simulink model "Diesel_Genset_Test_System_80kVA"  (Simulink 8.1)
settings: Solver=ode3  SolverMode=SingleTasking  StartTime=0.0  StopTime=30  FixedStep=Ts  RelTol=1e-3
PostLoadFcn:
  | Ts=50e-6;GenSelect='80kW';initGTS;
InitFcn:
  | Ts=50e-6;GenSelect='80kW';initGTS;
values from neighbouring files (symbols this model uses):
  GenPN = 4e6    (= 4000000)    [initGTS.m]
  GenVN = 13800    [initGTS.m]
  T3dend = [ 1.0000   -0.9913 ]    [initGTS.m]
  T3numd = [ 0    0.0087 ]    [initGTS.m]
  T4numd = [ 27.7778  -27.7237 ]    [initGTS.m]
undefined symbols (not defined in the file or in its folder): breakers_1ph_3ph, Diesel_Genset_lib, DiscIntNeverNeededParam, Gen_900kW_external_control, HIL_GenSet, Protection
libraries: powerlib x41, simulink x20, powerlib_extras x12, NG_Genset_lib x5, rtlab x2, cables_lib x2, powerlib_meascontrol x1
(part 2 of 2)

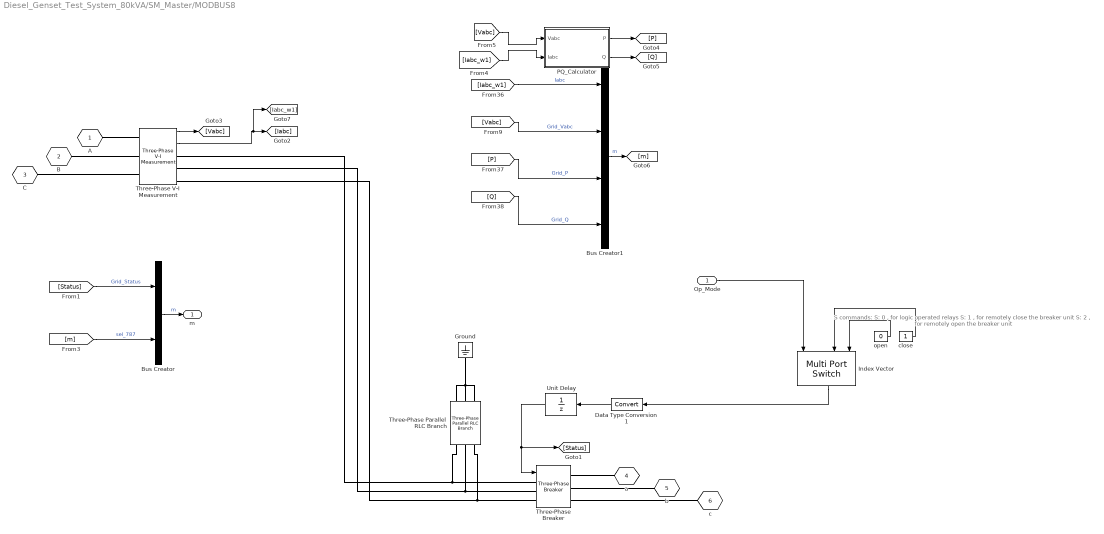
== system Diesel_Genset_Test_System_80kVA/SM_Master/MODBUS8 ==
  note: S commands:
      | S: 0 , for logic operated relays
      | S: 1 ,  for remotely close the breaker unit
      | S: 2 , for remotely open the breaker unit
  Op_Mode : Inport
  Bus Creator : BusCreator  Inputs=2
  Bus Creator1 : BusCreator
  Data Type Conversion1 : DataTypeConversion
  Ground : powerlib/Elements/Ground  LConnTagsString=a
  Index Vector : MultiPortSwitch  DataPortOrder=Zero-based contiguous  DataPortIndices={2,1,0}  zeroidx=on
  PQ_Calculator : Subsystem
  Three-Phase Parallel RLC Branch : powerlib/Elements/Three-Phase Parallel RLC Branch  LConnTagsString=A|B|C  RConnTagsString=A|B|C  BranchType=R  Resistance=10e6  Inductance=1e-3  Capacitance=1e-6  Measurements=None
  Three-Phase V-I Measurement : powerlib/Measurements/Three-Phase V-I Measurement  VoltageMeasurement=phase-to-ground  SetLabelV=off  LabelV=Vabc  Vpu=off  VpuLL=off  CurrentMeasurement=yes  SetLabelI=off  LabelI=Iabc  Ipu=off  Pbase=100e6  Vbase=500e3  OutputType=Complex  PhasorSimulation=off  PSBequivalent=0
  Three-Phase Breaker : powerlib/Elements/Three-Phase Breaker  InitialState=open  SwitchA=on  SwitchB=on  SwitchC=on  SwitchTimes="[1/60  5/60]"  External=on  BreakerResistance=1e-3  SnubberResistance=0  SnubberCapacitance=0  Measurements=None
  Unit Delay : UnitDelay  SampleTime=-1
  close : Constant
  open : Constant  Value=0
  A : PMIOPort  Tag=PMCPort  Port=1  Side=Left
  B : PMIOPort  Tag=PMCPort  Port=2  Side=Left
  C : PMIOPort  Tag=PMCPort  Port=3  Side=Left
  a : PMIOPort  Tag=PMCPort  Port=4  Side=Right
  b : PMIOPort  Tag=PMCPort  Port=5  Side=Right
  c : PMIOPort  Tag=PMCPort  Port=6  Side=Right
  m : Outport
  wires:
  [m] -> Bus Creator/2  "sel_787"
  Bus Creator/1 -> m/1  "m"
  [Status] -> Bus Creator/1  "Grid_Status"
  Unit Delay/1 -> [Status], Three-Phase Breaker/1
  Three-Phase V-I Measurement/1 -> [Vabc]
  Three-Phase V-I Measurement/2 -> [Iabc_w1], [Iabc]
  open/1 -> Index Vector/4
  close/1 -> Index Vector/3
  Index Vector/1 -> Data Type Conversion1/1
  Data Type Conversion1/1 -> Unit Delay/1
  Op_Mode/1 -> Index Vector/1
  [Q] -> Bus Creator1/4  "Grid_Q"
  [P] -> Bus Creator1/3  "Grid_P"
  [Vabc] -> Bus Creator1/2  "Grid_Vabc"
  [Iabc_w1] -> Bus Creator1/1  "Iabc"
  Bus Creator1/1 -> [m]  "m"
  [Vabc] -> PQ_Calculator/1(Vabc)
  [Iabc_w1] -> PQ_Calculator/2(Iabc)
  PQ_Calculator/1(P) -> [P]
  PQ_Calculator/2(Q) -> [Q]
  connections:
  Three-Phase V-I Measurement/RConn1 -- Three-Phase Parallel RLC Branch/RConn1 -- Three-Phase Breaker/LConn1
  Three-Phase V-I Measurement/RConn2 -- Three-Phase Parallel RLC Branch/RConn2 -- Three-Phase Breaker/LConn2
  Three-Phase V-I Measurement/RConn3 -- Three-Phase Parallel RLC Branch/RConn3 -- Three-Phase Breaker/LConn3
  Three-Phase Breaker/RConn2 -- b/RConn1
  Three-Phase Breaker/RConn3 -- c/RConn1
  Three-Phase V-I Measurement/LConn1 -- A/RConn1
  a/RConn1 -- Three-Phase Breaker/RConn1
  C/RConn1 -- Three-Phase V-I Measurement/LConn3
  B/RConn1 -- Three-Phase V-I Measurement/LConn2
  Ground/LConn1 -- Three-Phase Parallel RLC Branch/LConn2 -- Three-Phase Parallel RLC Branch/LConn3 -- Three-Phase Parallel RLC Branch/LConn1

== system Diesel_Genset_Test_System_80kVA/SC_Console/Woodward/16Din/16Dout GR3 ==
  Bus Creator2 : BusCreator  Inputs=8
  Closed 3 - 26 s1 : simulink/Sources/Repeating Sequence Stair  OutValues=[1 1 1 0 0 0 0 0 0 0 0 0 0 0 0 0 0 0 0 0 0 0 0 0 0 0 1 1 1 1 1 ]  tsamp=[1 Ts]  OutMin=[]  OutMax=[]  OutDataTypeStr=double  OutputDataTypeScalingMode=double  OutDataType=fixdt(0,8)  ConRadixGroup=Best Precision: Vector-wise  OutScaling=2^-12
  Constant5 : Constant  Value=0
  Constant6 : Constant
  Constant7 : Constant  Value=0
  Constant8 : Constant
  DO10_ExtAlarm : ManualSwitch  CurrentSetting=0
  DO11_EnableMCB : ManualSwitch  CurrentSetting=0
  DO12_MCBOpen : ManualSwitch  CurrentSetting=0
  DO13_GCBOpen : ManualSwitch  CurrentSetting=0
  DO14 : ManualSwitch  CurrentSetting=0
  DO15 : ManualSwitch  CurrentSetting=0
  DO8_Estop : ManualSwitch
  DO9_Start/Auto : ManualSwitch  CurrentSetting=0
  Dout : Outport
  wires:
  Bus Creator2/1 -> Dout/1  "DO"
  Constant6/1 -> DO9_Start/Auto/1, DO11_EnableMCB/1, DO10_ExtAlarm/1, DO8_Estop/1
  Constant5/1 -> DO9_Start/Auto/2, DO11_EnableMCB/2, DO10_ExtAlarm/2, DO8_Estop/2
  DO8_Estop/1 -> Bus Creator2/1  "Gen_Estop"
  DO9_Start/Auto/1 -> Bus Creator2/2  "Gen_StartAuto"
  DO10_ExtAlarm/1 -> Bus Creator2/3  "Gen_ExtAlarm"
  DO11_EnableMCB/1 -> Bus Creator2/4  "Gen_EnableMCB"
  Constant8/1 -> DO14/1, DO15/1, DO13_GCBOpen/1, DO12_MCBOpen/1
  Constant7/1 -> DO14/2, DO15/2, DO13_GCBOpen/2, DO12_MCBOpen/2
  DO12_MCBOpen/1 -> Bus Creator2/5  "Gen_MCBOpen"
  DO14/1 -> Bus Creator2/7  "Gen_DI11_MCB_Busbar"
  DO15/1 -> Bus Creator2/8  "Gen_DI12_GCB_Busbar"
  Closed 3 - 26 s1/1 -> Bus Creator2/6  "Gen_GCBOpen"

== system Diesel_Genset_Test_System_80kVA/SM_Master/80kVA_Diesel_Generator/DIO - Woodward ==
  note: These are the inputs to
      | Woodward
  Din_sim : Inport
  Gen2 MCB Status : Inport  Port=2
  Add2 : Sum
  Bus Selector2 : BusSelector  OutputSignals=Gen_Estop,Gen_StartAuto,Gen_ExtAlarm,Gen_EnableMCB,Gen_MCBOpen,Gen_GCBOpen,Gen_DI11_MCB_Busbar,Gen_DI12_GCB_Busbar
  Constant3 : Constant
  Data Type Conversion : DataTypeConversion  OutDataTypeStr=double
  Logical Operator1 : Logic  Operator=NOT  AllPortsSameDT=off  OutDataTypeStr=boolean
  Mux1 : Mux  Inputs=8
  Gen2 GCB : Outport
  wires:
  Mux1/1 -> ?  "DI_CH08-15"
  Add2/1 -> Gen2 GCB/1
  Constant3/1 -> Add2/2
  Bus Selector2/1 -> Mux1/1  "<Gen_Estop>"
  Bus Selector2/2 -> Mux1/2  "<Gen_StartAuto>"
  Bus Selector2/3 -> Mux1/3  "<Gen_ExtAlarm>"
  Bus Selector2/4 -> Mux1/4  "<Gen_EnableMCB>"
  Bus Selector2/5 -> ?  "<Gen_MCBOpen>"
  Bus Selector2/6 -> Add2/1, Mux1/6  "<Gen_GCBOpen>"
  Din_sim/1 -> Bus Selector2/1
  Bus Selector2/7 -> ?  "<Gen_DI11_MCB_Busbar>"
  Gen2 MCB Status/1 -> Mux1/7, Logical Operator1/1
  Bus Selector2/8 -> Mux1/8  "<Gen_DI12_GCB_Busbar>"
  Logical Operator1/1 -> Data Type Conversion/1
  Data Type Conversion/1 -> Mux1/5

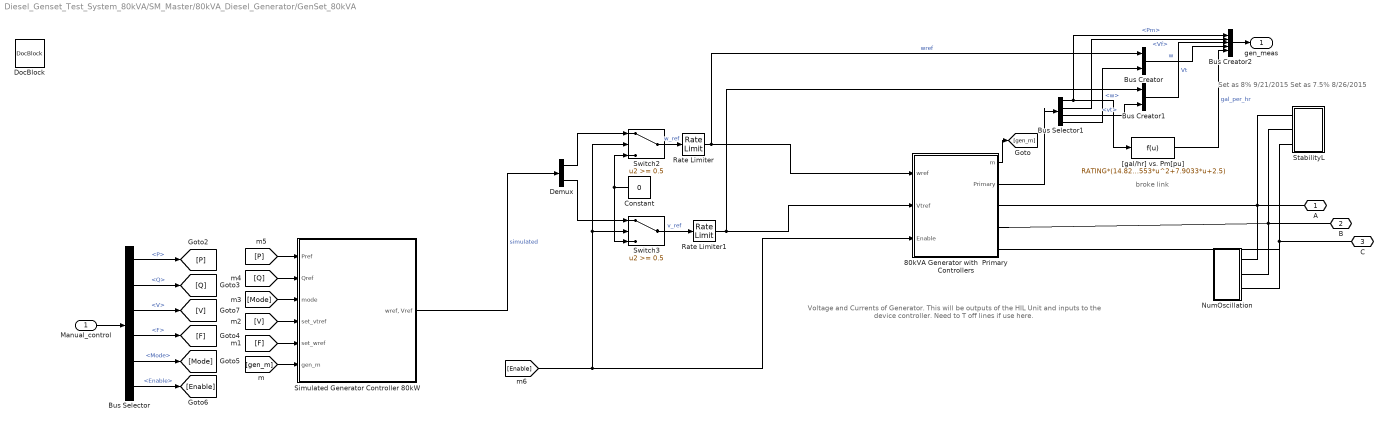
== system Diesel_Genset_Test_System_80kVA/SM_Master/80kVA_Diesel_Generator/GenSet_80kVA ==
  note: broke link
  note: Set as 8% 9/21/2015
      | Set as 7.5% 8/26/2015
  note: Voltage and Currents of Generator.
      | This will be outputs of the HIL Unit
      | and inputs to the device controller.
      | Need to T off lines if use here.
  Manual_control : Inport
  80kVA Generator with  Primary Controllers : Subsystem
  Bus Creator : BusCreator  Inputs=2
  Bus Creator1 : BusCreator  Inputs=2
  Bus Creator2 : BusCreator  Inputs=5
  Bus Selector : BusSelector  OutputSignals=P,Q,V,F,Mode,Enable
  Bus Selector1 : BusSelector  OutputSignals=Pm,Vf,vt,w
  Constant : Constant  Value=0
  Demux : Demux  Outputs=2
  DocBlock : simulink/Model-Wide Utilities/DocBlock  DocumentType=Text
  NumOscillation : Subsystem
  Rate Limiter : RateLimiter  RisingSlewLimit=0.5  FallingSlewLimit=-0.5  SampleTimeMode=inherited
  Rate Limiter1 : RateLimiter  RisingSlewLimit=0.5  FallingSlewLimit=-0.5  SampleTimeMode=inherited
  Simulated Generator Controller 80kW : Subsystem
  StabilityL : Subsystem  mask{v=GenVN, kVA=GenPN*0.2/1000, pf=1}
  Switch2 : Switch  Threshold=0.5
  Switch3 : Switch  Threshold=0.5
  "[gal/hr] vs. Pm[pu]" : Fcn  Expr=RATING*(14.827*u^4-27.253*u^3+15.553*u^2+7.9033*u+2.5)  mask{RATING=4}
      mask prompts: RATING "Rating [MW]"
      mask help: This block computes the gal/hr vs Pm[pu] of a generator of a given rating [MW].
  A : PMIOPort  Port=1  Side=Right
  B : PMIOPort  Port=2  Side=Right
  C : PMIOPort  Port=3  Side=Right
  gen_meas : Outport
  wires:
  "[gal/hr] vs. Pm[pu]"/1 -> Bus Creator2/5  "gal_per_hr"
  Rate Limiter1/1 -> Bus Creator1/1, 80kVA Generator with  Primary Controllers/2(Vtref)
  Rate Limiter/1 -> Bus Creator/1, 80kVA Generator with  Primary Controllers/1(wref)  "wref"
  Bus Creator2/1 -> gen_meas/1
  Bus Creator/1 -> Bus Creator2/4  "w"
  Bus Creator1/1 -> Bus Creator2/3  "Vt"
  Bus Selector1/1 -> "[gal/hr] vs. Pm[pu]"/1, Bus Creator2/1  "<Pm>"
  Bus Selector1/2 -> Bus Creator2/2  "<Vf>"
  Bus Selector1/4 -> Bus Creator/2  "<w>"
  Bus Selector1/3 -> Bus Creator1/2  "<vt>"
  Switch3/1 -> Rate Limiter1/1  "v_ref"
  Constant/1 -> Switch2/3, Switch3/3
  Demux/2 -> Switch3/1
  Demux/1 -> Switch2/1
  Switch2/1 -> Rate Limiter/1  "w_ref"
  [Enable] -> Switch3/2, Switch2/2, 80kVA Generator with  Primary Controllers/3(Enable)
  80kVA Generator with  Primary Controllers/2(Primary) -> Bus Selector1/1
  Bus Selector/6 -> [Enable]  "<Enable>"
  80kVA Generator with  Primary Controllers/1(m) -> [gen_m]
  Simulated Generator Controller 80kW/1("wref, Vref") -> Demux/1  "simulated"
  Manual_control/1 -> Bus Selector/1
  Bus Selector/1 -> [P]  "<P>"
  Bus Selector/2 -> [Q]  "<Q>"
  Bus Selector/3 -> [V]  "<V>"
  Bus Selector/4 -> [F]  "<F>"
  Bus Selector/5 -> [Mode]  "<Mode>"
  [gen_m] -> Simulated Generator Controller 80kW/6(gen_m)
  [P] -> Simulated Generator Controller 80kW/1(Pref)
  [Q] -> Simulated Generator Controller 80kW/2(Qref)
  [Mode] -> Simulated Generator Controller 80kW/3(mode)
  [V] -> Simulated Generator Controller 80kW/4(set_vtref)
  [F] -> Simulated Generator Controller 80kW/5(set_wref)
  connections:
  NumOscillation/LConn3 -- 80kVA Generator with  Primary Controllers/RConn3 -- C/RConn1 -- StabilityL/LConn3
  NumOscillation/LConn2 -- B/RConn1 -- 80kVA Generator with  Primary Controllers/RConn2 -- StabilityL/LConn2
  NumOscillation/LConn1 -- 80kVA Generator with  Primary Controllers/RConn1 -- A/RConn1 -- StabilityL/LConn1

== system Diesel_Genset_Test_System_80kVA/SM_Master/MODBUS1/PQ_Calculator ==
  Vabc : Inport
  Iabc : Inport  Port=2
  3-phase  Instantaneous  Active & Reactive Power : powerlib_extras/Measurements/3-phase  Instantaneous  Active & Reactive Power
  Demux : Demux  Outputs=2
  Discrete  Mean value2 : powerlib_extras/Discrete Measurements/Discrete  Mean value  Freq=60  Vinit=0  Ts=Ts
  P : Outport
  Q : Outport  Port=2
  wires:
  3-phase  Instantaneous  Active & Reactive Power/1 -> Discrete  Mean value2/1
  Discrete  Mean value2/1 -> Demux/1
  Vabc/1 -> 3-phase  Instantaneous  Active & Reactive Power/1
  Iabc/1 -> 3-phase  Instantaneous  Active & Reactive Power/2
  Demux/1 -> P/1  "P"
  Demux/2 -> Q/1  "Q"

== system Diesel_Genset_Test_System_80kVA/SM_Master/MODBUS2/PQ_Calculator ==
  Vabc : Inport
  Iabc : Inport  Port=2
  3-phase  Instantaneous  Active & Reactive Power : powerlib_extras/Measurements/3-phase  Instantaneous  Active & Reactive Power
  Demux : Demux  Outputs=2
  Discrete  Mean value2 : powerlib_extras/Discrete Measurements/Discrete  Mean value  Freq=60  Vinit=0  Ts=Ts
  P : Outport
  Q : Outport  Port=2
  wires:
  3-phase  Instantaneous  Active & Reactive Power/1 -> Discrete  Mean value2/1
  Discrete  Mean value2/1 -> Demux/1
  Vabc/1 -> 3-phase  Instantaneous  Active & Reactive Power/1
  Iabc/1 -> 3-phase  Instantaneous  Active & Reactive Power/2
  Demux/1 -> P/1  "P"
  Demux/2 -> Q/1  "Q"

== system Diesel_Genset_Test_System_80kVA/SM_Master/MODBUS4/PQ_Calculator ==
  Vabc : Inport
  Iabc : Inport  Port=2
  3-phase  Instantaneous  Active & Reactive Power : powerlib_extras/Measurements/3-phase  Instantaneous  Active & Reactive Power
  Demux : Demux  Outputs=2
  Discrete  Mean value2 : powerlib_extras/Discrete Measurements/Discrete  Mean value  Freq=60  Vinit=0  Ts=Ts
  P : Outport
  Q : Outport  Port=2
  wires:
  3-phase  Instantaneous  Active & Reactive Power/1 -> Discrete  Mean value2/1
  Discrete  Mean value2/1 -> Demux/1
  Vabc/1 -> 3-phase  Instantaneous  Active & Reactive Power/1
  Iabc/1 -> 3-phase  Instantaneous  Active & Reactive Power/2
  Demux/1 -> P/1  "P"
  Demux/2 -> Q/1  "Q"

== system Diesel_Genset_Test_System_80kVA/SM_Master/MODBUS5/PQ_Calculator ==
  Vabc : Inport
  Iabc : Inport  Port=2
  3-phase  Instantaneous  Active & Reactive Power : powerlib_extras/Measurements/3-phase  Instantaneous  Active & Reactive Power
  Demux : Demux  Outputs=2
  Discrete  Mean value2 : powerlib_extras/Discrete Measurements/Discrete  Mean value  Freq=60  Vinit=0  Ts=Ts
  P : Outport
  Q : Outport  Port=2
  wires:
  3-phase  Instantaneous  Active & Reactive Power/1 -> Discrete  Mean value2/1
  Discrete  Mean value2/1 -> Demux/1
  Vabc/1 -> 3-phase  Instantaneous  Active & Reactive Power/1
  Iabc/1 -> 3-phase  Instantaneous  Active & Reactive Power/2
  Demux/1 -> P/1  "P"
  Demux/2 -> Q/1  "Q"

== system Diesel_Genset_Test_System_80kVA/SM_Master/MODBUS6/PQ_Calculator ==
  Vabc : Inport
  Iabc : Inport  Port=2
  3-phase  Instantaneous  Active & Reactive Power : powerlib_extras/Measurements/3-phase  Instantaneous  Active & Reactive Power
  Demux : Demux  Outputs=2
  Discrete  Mean value2 : powerlib_extras/Discrete Measurements/Discrete  Mean value  Freq=60  Vinit=0  Ts=Ts
  P : Outport
  Q : Outport  Port=2
  wires:
  3-phase  Instantaneous  Active & Reactive Power/1 -> Discrete  Mean value2/1
  Discrete  Mean value2/1 -> Demux/1
  Vabc/1 -> 3-phase  Instantaneous  Active & Reactive Power/1
  Iabc/1 -> 3-phase  Instantaneous  Active & Reactive Power/2
  Demux/1 -> P/1  "P"
  Demux/2 -> Q/1  "Q"

== system Diesel_Genset_Test_System_80kVA/SM_Master/MODBUS8/PQ_Calculator ==
  Vabc : Inport
  Iabc : Inport  Port=2
  3-phase  Instantaneous  Active & Reactive Power : powerlib_extras/Measurements/3-phase  Instantaneous  Active & Reactive Power
  Demux : Demux  Outputs=2
  Discrete  Mean value2 : powerlib_extras/Discrete Measurements/Discrete  Mean value  Freq=60  Vinit=0  Ts=Ts
  P : Outport
  Q : Outport  Port=2
  wires:
  3-phase  Instantaneous  Active & Reactive Power/1 -> Discrete  Mean value2/1
  Discrete  Mean value2/1 -> Demux/1
  Vabc/1 -> 3-phase  Instantaneous  Active & Reactive Power/1
  Iabc/1 -> 3-phase  Instantaneous  Active & Reactive Power/2
  Demux/1 -> P/1  "P"
  Demux/2 -> Q/1  "Q"

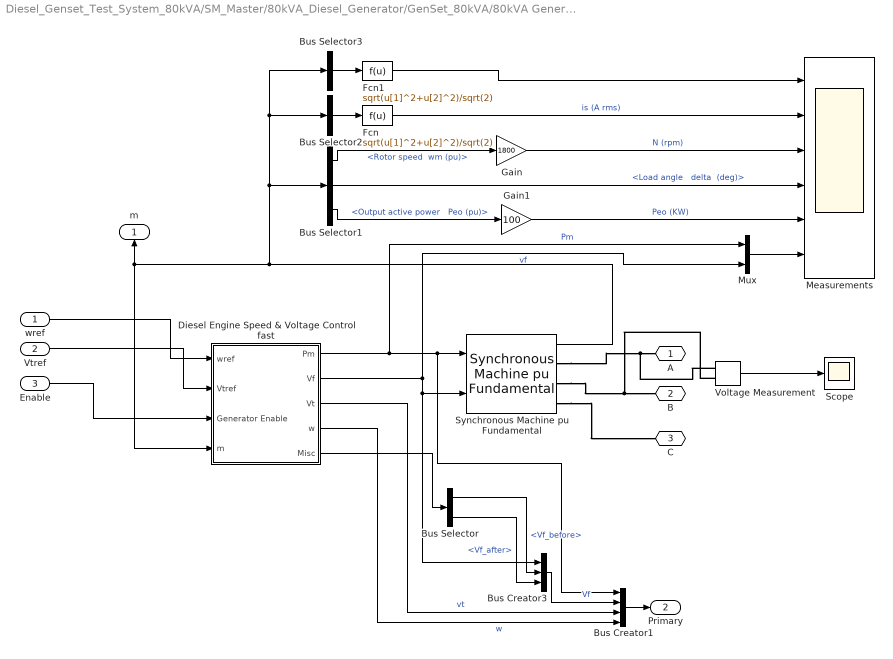
== system Diesel_Genset_Test_System_80kVA/SM_Master/80kVA_Diesel_Generator/GenSet_80kVA/80kVA Generator with  Primary Controllers ==
  wref : Inport
  Vtref : Inport  Port=2
  Enable : Inport  Port=3
  Bus Creator1 : BusCreator
  Bus Creator3 : BusCreator  Inputs=3
  Bus Selector : BusSelector  OutputSignals=Vf_before,Vf_after
  Bus Selector1 : BusSelector  OutputSignals="Mechanical.Rotor speed  wm (pu),Load angle   delta  (deg),Output active power   Peo (pu)"
  Bus Selector2 : BusSelector  OutputSignals="dq0 components.Stator current  iq (pu),dq0 components.Stator current  id (pu)"  OutputAsBus=on
  Bus Selector3 : BusSelector  OutputSignals="dq0 components.Stator voltage  vq (pu),dq0 components.Stator voltage  vd (pu)"  OutputAsBus=on
  Diesel Engine Speed & Voltage Control fast : Subsystem
  Fcn : Fcn  Expr=sqrt(u[1]^2+u[2]^2)/sqrt(2)
  Fcn1 : Fcn  Expr=sqrt(u[1]^2+u[2]^2)/sqrt(2)
  Gain : Gain  Gain=1800  SaturateOnIntegerOverflow=on  OutDataTypeStr=Inherit: Same as input  ParamDataTypeStr=Inherit: Same as input
  Gain1 : Gain  Gain=100  SaturateOnIntegerOverflow=on  OutDataTypeStr=Inherit: Same as input  ParamDataTypeStr=Inherit: Same as input
  Measurements : Scope  NumInputPorts=6
      settings: TickLabels=on  TimeRange=3  YMin=0.1~0~1500~-200~-400~-1  YMax=0.8~8~2100~200~300~5  SaveName=is
  Mux : Mux  Inputs=2
  Scope : Scope
      settings: YMin=-750  YMax=750  SaveName=ScopeData12  Decimation=10
  Synchronous Machine pu Fundamental : powerlib/Machines/Synchronous Machine pu Fundamental  PresetModel=No  MechanicalLoad=Mechanical power Pm  ShowDetailedParameters=on  RotorType=Salient-pole  NominalParameters=[80e3 480 60]  Stator=[0.02599 0.07 2.25 0.99]  Field=[0.016 0.2092]  Dampers2=[0.0652, 0.5134, 0.0287, 0.2553, 7.765e-3, 0.9167 ]  Dampers1=[0.2047 0.6524 0.04286 0.06387]  Mechanical=[0.1268 0.02132 2]  PolePairs=2  InitialConditions="[ -99  0  0  0  0  0  0  0  0 ]"  SetSaturation=off  Saturation=[0.6404,0.7127,0.8441,0.9214,0.9956,1.082,1.19,1.316,1.457;0.7,0.7698,0.8872,0.9466,0.9969,1.046,1.1,1.151,1.201]  Units=per unit fundamental parameters  LoadFlowParameters=[1,0,0,0,0]  TsPowergui=0  TsBlock=-1  IterativeModel=Forward Euler  BusType=swing  Pref=0  Qref=0  Qmin=-inf  Qmax=inf  PLF=0  QLF=0
  Voltage Measurement : powerlib/Measurements/Voltage Measurement  PhasorSimulation=off  OutputType=Complex  PSBequivalent=0
  A : PMIOPort  Port=1  Side=Right
  B : PMIOPort  Port=2  Side=Right
  C : PMIOPort  Port=3  Side=Right
  m : Outport
  Primary : Outport  Port=2
  wires:
  Bus Creator3/1 -> Bus Creator1/2  "Vf"
  Bus Selector/2 -> Bus Creator3/3  "<Vf_after>"
  Bus Selector/1 -> Bus Creator3/2  "<Vf_before>"
  Diesel Engine Speed & Voltage Control fast/5(Misc) -> Bus Selector/1
  Bus Creator1/1 -> Primary/1
  Diesel Engine Speed & Voltage Control fast/4(w) -> Bus Creator1/4  "w"
  Diesel Engine Speed & Voltage Control fast/3(Vt) -> Bus Creator1/3  "vt"
  Synchronous Machine pu Fundamental/1 -> Bus Selector1/1, Bus Selector2/1, Bus Selector3/1, Diesel Engine Speed & Voltage Control fast/4(m), m/1
  Enable/1 -> Diesel Engine Speed & Voltage Control fast/3(Generator Enable)
  Diesel Engine Speed & Voltage Control fast/1(Pm) -> Mux/1, Synchronous Machine pu Fundamental/1, Bus Creator1/1  "Pm"
  Diesel Engine Speed & Voltage Control fast/2(Vf) -> Synchronous Machine pu Fundamental/2, Bus Creator3/1, Mux/2  "vf"
  wref/1 -> Diesel Engine Speed & Voltage Control fast/1(wref)
  Vtref/1 -> Diesel Engine Speed & Voltage Control fast/2(Vtref)
  Fcn/1 -> Measurements/2  "is (A rms)"
  Bus Selector2/1 -> Fcn/1
  Gain/1 -> Measurements/3  "N (rpm)"
  Gain1/1 -> Measurements/5  "Peo (KW)"
  Bus Selector1/3 -> Gain1/1  "<Output active power   Peo (pu)>"
  Bus Selector1/2 -> Measurements/4  "<Load angle   delta  (deg)>"
  Bus Selector1/1 -> Gain/1  "<Rotor speed  wm (pu)>"
  Bus Selector3/1 -> Fcn1/1
  Fcn1/1 -> Measurements/1
  Mux/1 -> Measurements/6
  Voltage Measurement/1 -> Scope/1
  connections:
  Synchronous Machine pu Fundamental/RConn1 -- Voltage Measurement/LConn1 -- A/RConn1
  Synchronous Machine pu Fundamental/RConn2 -- Voltage Measurement/LConn2 -- B/RConn1
  Synchronous Machine pu Fundamental/RConn3 -- C/RConn1

== system Diesel_Genset_Test_System_80kVA/SM_Master/80kVA_Diesel_Generator/GenSet_80kVA/NumOscillation ==
  Ground2 : powerlib/Elements/Ground  LConnTagsString=a
  "RLC " : powerlib/Elements/Parallel RLC Branch  LConnTagsString=a  RConnTagsString=__new0  BranchType=R  Resistance=10e6  Inductance=inf  SetiL0=off  InitialCurrent=0  Capacitance=10e-6  Setx0=off  InitialVoltage=0  Measurements=None
  RLC1 : powerlib/Elements/Parallel RLC Branch  LConnTagsString=a  RConnTagsString=__new0  BranchType=R  Resistance=10e6  Inductance=inf  SetiL0=off  InitialCurrent=0  Capacitance=10e-6  Setx0=off  InitialVoltage=0  Measurements=None
  RLC2 : powerlib/Elements/Parallel RLC Branch  LConnTagsString=a  RConnTagsString=__new0  BranchType=R  Resistance=10e6  Inductance=inf  SetiL0=off  InitialCurrent=0  Capacitance=10e-6  Setx0=off  InitialVoltage=0  Measurements=None
  RLC3 : powerlib/Elements/Parallel RLC Branch  LConnTagsString=a  RConnTagsString=__new0  BranchType=R  Resistance=10e-3  Inductance=inf  SetiL0=off  InitialCurrent=0  Capacitance=0  Setx0=off  InitialVoltage=0  Measurements=None
  RLC4 : powerlib/Elements/Parallel RLC Branch  LConnTagsString=a  RConnTagsString=__new0  BranchType=R  Resistance=10e-3  Inductance=inf  SetiL0=off  InitialCurrent=0  Capacitance=0  Setx0=off  InitialVoltage=0  Measurements=None
  RLC5 : powerlib/Elements/Parallel RLC Branch  LConnTagsString=a  RConnTagsString=__new0  BranchType=R  Resistance=10e-3  Inductance=inf  SetiL0=off  InitialCurrent=0  Capacitance=0  Setx0=off  InitialVoltage=0  Measurements=None
  A : PMIOPort  Port=1  Side=Left
  B : PMIOPort  Port=2  Side=Left
  C : PMIOPort  Port=3  Side=Left
  connections:
  "RLC "/RConn1 -- RLC1/RConn1 -- Ground2/LConn1 -- RLC2/RConn1
  "RLC "/LConn1 -- RLC5/RConn1
  RLC1/LConn1 -- RLC4/RConn1
  RLC3/RConn1 -- RLC2/LConn1
  A/RConn1 -- RLC3/LConn1
  B/RConn1 -- RLC4/LConn1
  C/RConn1 -- RLC5/LConn1

== system Diesel_Genset_Test_System_80kVA/SM_Master/80kVA_Diesel_Generator/GenSet_80kVA/Simulated Generator Controller 80kW ==
  Pref : Inport
  Qref : Inport  Port=2
  mode : Inport  Port=3
  set_vtref : Inport  Port=4
  set_wref : Inport  Port=5
  gen_m : Inport  Port=6
  Bus Selector1 : BusSelector  OutputSignals="Output active power   Peo (pu),Output reactive power  Qeo (pu)"
  Compare To Constant : simulink/Logic and Bit Operations/Compare To Constant  relop=~=  const=1  OutDataTypeStr=boolean
  Demux : Demux  Outputs=2
  Multiport Switch : MultiPortSwitch  DiagnosticForDefault=Warning
  Mux1 : Mux  Inputs=2
  Mux2 : Mux  Inputs=2
  Mux3 : Mux  Inputs=2
  PQ control : Subsystem
  PV control : Subsystem
  Unit Delay : UnitDelay  SampleTime=-1
  "wref, Vref" : Outport
  wires:
  Multiport Switch/1 -> Unit Delay/1, "wref, Vref"/1
  mode/1 -> Compare To Constant/1, Multiport Switch/1
  Qref/1 -> PQ control/3(Q_ref (pu))
  set_wref/1 -> Mux3/1
  Bus Selector1/2 -> PQ control/4(Q (pu))  "<Output reactive power  Qeo (pu)>"
  Pref/1 -> PV control/1(P_ref (pu)), PQ control/1(P_ref (pu))
  Mux3/1 -> Multiport Switch/4
  Mux2/1 -> Multiport Switch/3
  Mux1/1 -> Multiport Switch/2
  set_vtref/1 -> Mux3/2, Mux2/2
  PV control/1(w_ref (pu)) -> Mux2/1
  PQ control/2(V_ref (pu)) -> Mux1/2
  PQ control/1(w_ref (pu)) -> Mux1/1
  gen_m/1 -> Bus Selector1/1
  Bus Selector1/1 -> PV control/2(P (pu)), PQ control/2(P (pu))  "<Output active power   Peo (pu)>"
  Compare To Constant/1 -> PQ control/5(Rst)
  Demux/1 -> PQ control/6(w_Rst)
  Demux/2 -> PQ control/7(V_Rst)
  Unit Delay/1 -> Demux/1

== system Diesel_Genset_Test_System_80kVA/SM_Master/80kVA_Diesel_Generator/GenSet_80kVA/StabilityL ==
  Constant Load : powerlib/Elements/Three-Phase Parallel RLC Load  LConnTagsString=A|B|C  Configuration=Y (grounded)  NominalVoltage=v  NominalFrequency=60  ActivePower=kVA*1E3*pf  InductivePower=kVA*1E3*sqrt(1-pf^2)  CapacitivePower=0  Measurements=None  LoadType=constant Z
  A : PMIOPort  Port=1  Side=Left
  B : PMIOPort  Port=2  Side=Left
  C : PMIOPort  Port=3  Side=Left
  connections:
  C/RConn1 -- Constant Load/LConn3
  B/RConn1 -- Constant Load/LConn2
  A/RConn1 -- Constant Load/LConn1

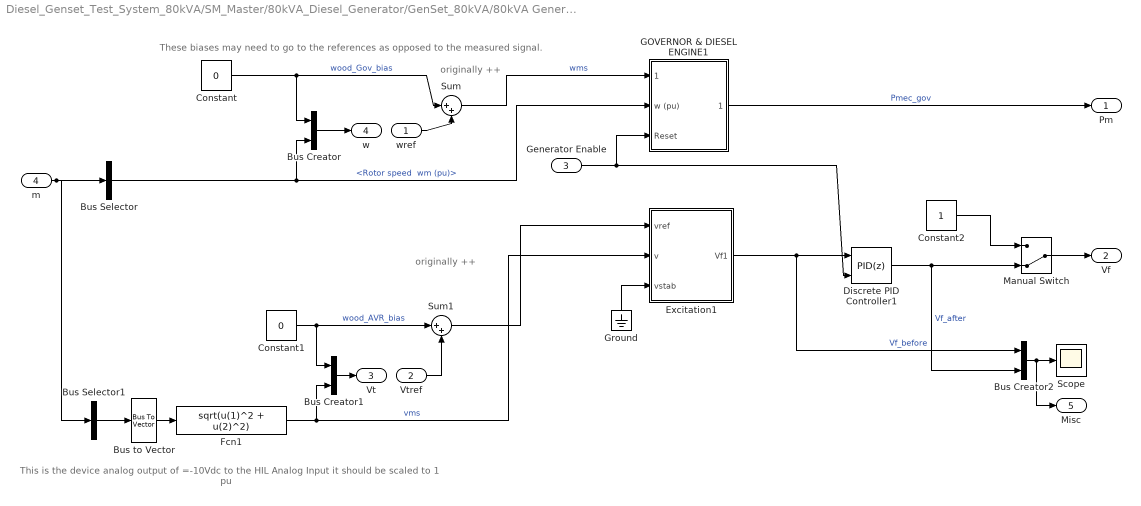
== system Diesel_Genset_Test_System_80kVA/SM_Master/80kVA_Diesel_Generator/GenSet_80kVA/80kVA Generator with  Primary Controllers/Diesel Engine Speed & Voltage Control fast ==
  note: originally ++
  note: originally ++
  note: These biases may need to
      | go to the references as opposed
      | to the measured signal.
  note: This is the device analog output of =-10Vdc to
      | the HIL Analog Input it should be scaled to 1 pu
  wref : Inport  SampleTime=Ts
  Vtref : Inport  Port=2  SampleTime=Ts
  Generator Enable : Inport  Port=3  SampleTime=Ts
  m : Inport  Port=4  SampleTime=Ts
  Bus Creator : BusCreator  Inputs=2
  Bus Creator1 : BusCreator  Inputs=2
  Bus Creator2 : BusCreator  Inputs=2
  Bus Selector : BusSelector  OutputSignals="Mechanical.Rotor speed  wm (pu)"
  Bus Selector1 : BusSelector  OutputSignals="dq0 components.Stator voltage  vd (pu),dq0 components.Stator voltage  vq (pu)"  OutputAsBus=on
  Bus to Vector : BusToVector
  Constant : Constant  Value=0
  Constant1 : Constant  Value=0
  Constant2 : Constant
  Discrete PID Controller1 : simulink/Continuous/PID Controller  Controller=PID  TimeDomain=Discrete-time  SampleTime=-1  IntegratorMethod=Forward Euler  FilterMethod=Forward Euler  Form=Parallel  P=1  I=0  D=0  N=100  InitialConditionSource=internal  InitialConditionForIntegrator=0  InitialConditionForFilter=0  ExternalReset=either  LimitOutput=on  UpperSaturationLimit=5  LowerSaturationLimit=-5  LinearizeAsGain=off  AntiWindupMode=none  Kb=1  TrackingMode=off  Kt=1  PParamMin=[]  PParamMax=[]  IParamMin=[]  IParamMax=[]  DParamMin=[]  DParamMax=[]  NParamMin=[]  NParamMax=[]  KbParamMin=[]  KbParamMax=[]  KtParamMin=[]  KtParamMax=[]  POutMin=[]  POutMax=[]  IOutMin=[]  IOutMax=[]  DOutMin=[]  DOutMax=[]  NOutMin=[]  NOutMax=[]  KbOutMin=[]  KbOutMax=[]  KtOutMin=[]  KtOutMax=[]  IntegratorOutMin=[]  IntegratorOutMax=[]  FilterOutMin=[]  FilterOutMax=[]  SumOutMin=[]  SumOutMax=[]  SumI1OutMin=[]  SumI1OutMax=[]  SumI2OutMin=[]  SumI2OutMax=[]  SumI3OutMin=[]  SumI3OutMax=[]  SumDOutMin=[]  SumDOutMax=[]  SaturationOutMin=[]  SaturationOutMax=[]  IntegratorContinuousStateAttributes=''  IntegratorStateMustResolveToSignalObject=off  IntegratorRTWStateStorageClass=Auto  FilterContinuousStateAttributes=''  FilterStateMustResolveToSignalObject=off  FilterRTWStateStorageClass=Auto
  Excitation1 : Subsystem  mask(Excitation System){tr=2e-3, reg=[ 100 20e-3 ], exc=[ 1 0.02 ], tgr=[ 1e-12 1e-12 ], damp=[0.03 1 ], sat=[], lim=[ 0 5 0 ], v0=[ 0 0 ]}
      mask prompts: tr "Low-pass filter time constant Tr:"; reg "Regulator gain and time constant [ Ka  Ta ]:"; exc "Exciter  [ Ke  Te ]:"; tgr "Transient gain reduction [ Tb  Tc ]:"; damp "Damping filter gain and time constant  [ Kf  Tf  ]:"; sat "Field saturation parameters [ A B ]:"; lim "Regulator output limits and gain [ Efmin  Efmax  Kp ]:"; v0 "Initial values of terminal voltage  and field voltage [ Vt0 Vf0 ] :"
      mask help:
      | Implements an IEEE type 1 synchronous machine voltage regulator combined
      | to an exciter.
      |
      | The output of the block is the field voltage vfd, in pu,  to be applied to the Vf
      | Simulink input of a Synchronous Machine block.
      |
      | Connect the Vd and Vq measurements signals of the Synchronous Machine block
      | (signals 9 and 10)  to  the Vd and Vq inputs of the Excitation System block.
      mask Help: helpview(psbhelp);
  Fcn1 : Fcn  Expr=sqrt(u(1)^2 + u(2)^2)
  GOVERNOR & DIESEL ENGINE1 : Subsystem  mask(Diesel Engine & Governor){K=1, Ta=[0.025 0.0009 0.00574], Tlim=[0 2], Td=0.024, Pm0=0.00005}
      mask prompts: K "Regulator gain K:"; Ta "Actuator time constants [T4 T5 T6] (s) :"; Tlim "Torque limits [Tmin Tmax] (pu) :"; Td "Engine time delay Td (s) :"; Pm0 "Initial value of mechanical power  Pm0 (pu) :"
      mask help:
      | This block implements a diesel engine and governor system:
      | 1st and 2nd inputs: Desired and actual speed (pu)
      | Output: Diesel engine mechanical power.Motor inertia should be combined with generator.
      |
      | Actuator transfer function :
      |      Ha= (1+T4.s) / [ (s (1+T5.s)(1+T6.s) ]
      | Motor :
      |      Time delay Td
      |
      | (See reference in Tutorial Session 5)
  Ground : Ground
  Manual Switch : ManualSwitch  CurrentSetting=0
  Scope : Scope
      settings: YMin=1.0475  YMax=1.08
  Sum : Sum  Inputs=|++
  Sum1 : Sum  Inputs=|++
  Pm : Outport
  Vf : Outport  Port=2
  Vt : Outport  Port=3
  w : Outport  Port=4
  Misc : Outport  Port=5
  wires:
  Sum/1 -> GOVERNOR & DIESEL ENGINE1/1(wref (pu))  "wms"
  wref/1 -> Sum/2
  Sum1/1 -> Excitation1/1(vref)
  Vtref/1 -> Sum1/2
  Constant1/1 -> Bus Creator1/1, Sum1/1  "wood_AVR_bias"
  Constant/1 -> Bus Creator/1, Sum/1  "wood_Gov_bias"
  Bus Creator2/1 -> Misc/1, Scope/1
  Discrete PID Controller1/1 -> Bus Creator2/2, Manual Switch/2  "Vf_after"
  Excitation1/1(Vf1) -> Bus Creator2/1, Discrete PID Controller1/1  "Vf_before"
  Bus Creator1/1 -> Vt/1
  Bus Creator/1 -> w/1
  Ground/1 -> Excitation1/3(vstab)
  Fcn1/1 -> Excitation1/2(v), Bus Creator1/2  "vms"
  Bus Selector/1 -> GOVERNOR & DIESEL ENGINE1/2(w (pu)), Bus Creator/2  "<Rotor speed  wm (pu)>"
  m/1 -> Bus Selector/1, Bus Selector1/1
  Bus Selector1/1 -> Bus to Vector/1
  Bus to Vector/1 -> Fcn1/1
  Generator Enable/1 -> Discrete PID Controller1/2, GOVERNOR & DIESEL ENGINE1/3(Reset)
  GOVERNOR & DIESEL ENGINE1/1(Pmec (pu)) -> Pm/1  "Pmec_gov"
  Constant2/1 -> Manual Switch/1
  Manual Switch/1 -> Vf/1

== system Diesel_Genset_Test_System_80kVA/SM_Master/80kVA_Diesel_Generator/GenSet_80kVA/Simulated Generator Controller 80kW/PQ control ==
  P_ref (pu) : Inport
  P (pu) : Inport  Port=2
  Q_ref (pu) : Inport  Port=3
  Q (pu) : Inport  Port=4
  Rst : Inport  Port=5
  w_Rst : Inport  Port=6
  V_Rst : Inport  Port=7
  Constant : Constant
  Discrete PID Controller : simulink/Continuous/PID Controller  Controller=PID  TimeDomain=Discrete-time  SampleTime=-1  IntegratorMethod=Forward Euler  FilterMethod=Forward Euler  Form=Parallel  P=0.025  I=1  D=0  N=10  InitialConditionSource=external  InitialConditionForIntegrator=0  InitialConditionForFilter=0  ExternalReset=level  LimitOutput=on  UpperSaturationLimit=1.15  LowerSaturationLimit=0.85  LinearizeAsGain=off  AntiWindupMode=back-calculation  Kb=1  TrackingMode=off  Kt=1  PParamMin=[]  PParamMax=[]  IParamMin=[]  IParamMax=[]  DParamMin=[]  DParamMax=[]  NParamMin=[]  NParamMax=[]  KbParamMin=[]  KbParamMax=[]  KtParamMin=[]  KtParamMax=[]  POutMin=[]  POutMax=[]  IOutMin=[]  IOutMax=[]  DOutMin=[]  DOutMax=[]  NOutMin=[]  NOutMax=[]  KbOutMin=[]  KbOutMax=[]  KtOutMin=[]  KtOutMax=[]  IntegratorOutMin=[]  IntegratorOutMax=[]  FilterOutMin=[]  FilterOutMax=[]  SumOutMin=[]  SumOutMax=[]  SumI1OutMin=[]  SumI1OutMax=[]  SumI2OutMin=[]  SumI2OutMax=[]  SumI3OutMin=[]  SumI3OutMax=[]  SumDOutMin=[]  SumDOutMax=[]  SaturationOutMin=[]  SaturationOutMax=[]  IntegratorContinuousStateAttributes=''  IntegratorStateMustResolveToSignalObject=off  IntegratorRTWStateStorageClass=Auto  FilterContinuousStateAttributes=''  FilterStateMustResolveToSignalObject=off  FilterRTWStateStorageClass=Auto
  Discrete PID Controller1 : simulink/Continuous/PID Controller  Controller=PID  TimeDomain=Discrete-time  SampleTime=-1  IntegratorMethod=Forward Euler  FilterMethod=Forward Euler  Form=Parallel  P=0.02  I=1.5  D=0  N=10  InitialConditionSource=external  InitialConditionForIntegrator=0  InitialConditionForFilter=0  ExternalReset=level  LimitOutput=on  UpperSaturationLimit=1.15  LowerSaturationLimit=0.85  LinearizeAsGain=off  AntiWindupMode=back-calculation  Kb=1  TrackingMode=off  Kt=1  PParamMin=[]  PParamMax=[]  IParamMin=[]  IParamMax=[]  DParamMin=[]  DParamMax=[]  NParamMin=[]  NParamMax=[]  KbParamMin=[]  KbParamMax=[]  KtParamMin=[]  KtParamMax=[]  POutMin=[]  POutMax=[]  IOutMin=[]  IOutMax=[]  DOutMin=[]  DOutMax=[]  NOutMin=[]  NOutMax=[]  KbOutMin=[]  KbOutMax=[]  KtOutMin=[]  KtOutMax=[]  IntegratorOutMin=[]  IntegratorOutMax=[]  FilterOutMin=[]  FilterOutMax=[]  SumOutMin=[]  SumOutMax=[]  SumI1OutMin=[]  SumI1OutMax=[]  SumI2OutMin=[]  SumI2OutMax=[]  SumI3OutMin=[]  SumI3OutMax=[]  SumDOutMin=[]  SumDOutMax=[]  SaturationOutMin=[]  SaturationOutMax=[]  IntegratorContinuousStateAttributes=''  IntegratorStateMustResolveToSignalObject=off  IntegratorRTWStateStorageClass=Auto  FilterContinuousStateAttributes=''  FilterStateMustResolveToSignalObject=off  FilterRTWStateStorageClass=Auto
  Manual Switch : ManualSwitch  CurrentSetting=0
  Mux : Mux  Inputs=2
  Mux1 : Mux  Inputs=2
  Scope : Scope  NumInputPorts=5
      settings: YMin=0.265~0.996~-0.125~1.15~-1  YMax=0.325~1.01~0.15~1.15~1  SaveName=ScopeData8  Decimation=100
  Scope1 : Scope  NumInputPorts=5
      settings: YMin=1.03~1.15~-1~-1~-1  YMax=1.0475~1.15~1~1~1  SaveName=ScopeData9  Decimation=100
  Sum : Sum  Inputs=|-+
  Sum1 : Sum  Inputs=|-+
  w_ref (pu) : Outport
  V_ref (pu) : Outport  Port=2
  wires:
  Q_ref (pu)/1 -> Mux1/1, Sum1/2  "ref"
  Discrete PID Controller1/1 -> Manual Switch/2, Scope/4  "v"
  Q (pu)/1 -> Mux1/2, Sum1/1  "pu"
  Sum1/1 -> Discrete PID Controller1/1  "dq"
  P_ref (pu)/1 -> Mux/1, Sum/2
  Discrete PID Controller/1 -> Scope/2, w_ref (pu)/1
  P (pu)/1 -> Mux/2, Sum/1
  Sum/1 -> Discrete PID Controller/1
  Mux/1 -> Scope/1
  Rst/1 -> Discrete PID Controller/2, Discrete PID Controller1/2, Scope/5
  Mux1/1 -> Scope/3
  V_Rst/1 -> Scope1/2, Discrete PID Controller1/4, Discrete PID Controller1/3
  w_Rst/1 -> Scope1/1, Discrete PID Controller/3, Discrete PID Controller/4
  Manual Switch/1 -> V_ref (pu)/1
  Constant/1 -> Manual Switch/1

== system Diesel_Genset_Test_System_80kVA/SM_Master/80kVA_Diesel_Generator/GenSet_80kVA/Simulated Generator Controller 80kW/PV control ==
  P_ref (pu) : Inport
  P (pu) : Inport  Port=2
  Discrete PID Controller : simulink/Continuous/PID Controller  Controller=PID  TimeDomain=Discrete-time  SampleTime=-1  IntegratorMethod=Forward Euler  FilterMethod=Forward Euler  Form=Parallel  P=0.025  I=1  D=0  N=10  InitialConditionSource=internal  InitialConditionForIntegrator=0  InitialConditionForFilter=0  ExternalReset=none  LimitOutput=on  UpperSaturationLimit=1.15  LowerSaturationLimit=0.85  LinearizeAsGain=off  AntiWindupMode=back-calculation  Kb=1  TrackingMode=off  Kt=1  PParamMin=[]  PParamMax=[]  IParamMin=[]  IParamMax=[]  DParamMin=[]  DParamMax=[]  NParamMin=[]  NParamMax=[]  KbParamMin=[]  KbParamMax=[]  KtParamMin=[]  KtParamMax=[]  POutMin=[]  POutMax=[]  IOutMin=[]  IOutMax=[]  DOutMin=[]  DOutMax=[]  NOutMin=[]  NOutMax=[]  KbOutMin=[]  KbOutMax=[]  KtOutMin=[]  KtOutMax=[]  IntegratorOutMin=[]  IntegratorOutMax=[]  FilterOutMin=[]  FilterOutMax=[]  SumOutMin=[]  SumOutMax=[]  SumI1OutMin=[]  SumI1OutMax=[]  SumI2OutMin=[]  SumI2OutMax=[]  SumI3OutMin=[]  SumI3OutMax=[]  SumDOutMin=[]  SumDOutMax=[]  SaturationOutMin=[]  SaturationOutMax=[]  IntegratorContinuousStateAttributes=''  IntegratorStateMustResolveToSignalObject=off  IntegratorRTWStateStorageClass=Auto  FilterContinuousStateAttributes=''  FilterStateMustResolveToSignalObject=off  FilterRTWStateStorageClass=Auto
  Sum : Sum  Inputs=|-+
  w_ref (pu) : Outport
  wires:
  Sum/1 -> Discrete PID Controller/1
  P (pu)/1 -> Sum/1
  Discrete PID Controller/1 -> w_ref (pu)/1
  P_ref (pu)/1 -> Sum/2

== system Diesel_Genset_Test_System_80kVA/SM_Master/80kVA_Diesel_Generator/GenSet_80kVA/80kVA Generator with  Primary Controllers/Diesel Engine Speed & Voltage Control fast/Excitation1 ==
  note: link disabled
  note: link disabled
  vref : Inport
  v : Inport  Port=2
  vstab : Inport  Port=3
  Damping kf.s / (tf.s +1) : Subsystem
  Exciter  1 / (te.s + ke) : Subsystem
  Lead Lag Compensator tc.s+1 / tb.s+1 : NG_Genset_lib/NG Genset 3.5MVA/3.5MVA Generator with  Primary Controllers1/NG Engine Speed & Voltage Control fast/Excitation1/Lead Lag Compensator tc.s+1 // tb.s+1  T1=tgr(2)  T2=tgr(1)  V_Init=exc(1)*v0(2)/reg(1)  Ts=Ts
  Low Pass Filter 1 / (tr.s +1) (with IC) : NG_Genset_lib/NG Genset 3.5MVA/3.5MVA Generator with  Primary Controllers1/NG Engine Speed & Voltage Control fast/Excitation1/Low Pass Filter 1 // (tr.s +1) (with IC)  FilterType=Lowpass  Tc=tr  Ts=Ts  Initialize=on  Vac_Init=[0 0 60]  Vdc_Init=v0(1)  PlotResponse=off  param1=[1 500 0.1]
  Main Regulator ka / (ta.s +1) : Subsystem
  Mean : powerlib_meascontrol/Measurements/Mean  Freq=60  Vinit=v0(1)  Ts=Ts
  Mux : Mux  Inputs=3
  Mux1 : Mux  Inputs=2
  Scope : Scope  NumInputPorts=4
      settings: TimeRange=6  YMin=0.955~0~2.9~2.91  YMax=1~3~2.97~2.96  SaveName=ScopeData3  Decimation=10
  Sum : Sum  Inputs=++-+-  SaturateOnIntegerOverflow=on  InputSameDT=on  OutDataTypeStr=Inherit: Same as first input
  Unit Delay1 : UnitDelay  SampleTime=Ts
  Unit Delay2 : UnitDelay  InitialCondition=v0(2)  SampleTime=Ts
  Vf0 / ka : Constant  Value=v0(2)/reg(1)
  proportional saturation : Subsystem
  Vf1 : Outport  InitialOutput=0
  wires:
  Unit Delay2/1 -> Vf1/1
  Unit Delay1/1 -> Sum/5
  proportional saturation/1(Ef) -> Scope/3, Exciter  1 / (te.s + ke)/1(In)
  Lead Lag Compensator tc.s+1 / tb.s+1/1 -> Main Regulator ka / (ta.s +1)/1(In)
  Sum/1 -> Mux1/1, Lead Lag Compensator tc.s+1 / tb.s+1/1
  vref/1 -> Mux/1, Sum/1
  vstab/1 -> Sum/4
  v/1 -> Mean/1, Mux/2, Low Pass Filter 1 / (tr.s +1) (with IC)/1
  Vf0 / ka/1 -> Sum/2
  Main Regulator ka / (ta.s +1)/1(Out) -> Mux1/2, proportional saturation/1(Efd)
  Damping kf.s / (tf.s +1)/1(Out) -> Unit Delay1/1
  Exciter  1 / (te.s + ke)/1(Out) -> Unit Delay2/1, Scope/4, Damping kf.s / (tf.s +1)/1(In)
  Mux/1 -> Scope/1
  Mux1/1 -> Scope/2
  Low Pass Filter 1 / (tr.s +1) (with IC)/1 -> Mux/3, proportional saturation/2(Vtf), Sum/3

== system Diesel_Genset_Test_System_80kVA/SM_Master/80kVA_Diesel_Generator/GenSet_80kVA/80kVA Generator with  Primary Controllers/Diesel Engine Speed & Voltage Control fast/GOVERNOR & DIESEL ENGINE1 ==
  note: ACTUATOR
  wref (pu) : Inport
  w (pu) : Inport  Port=2
  Reset : Inport  Port=3
  Damping due to pumping losses : Gain  Gain=0.3
  Discrete PID Controller : simulink/Continuous/PID Controller  Controller=PD  TimeDomain=Discrete-time  SampleTime=-1  IntegratorMethod=Forward Euler  FilterMethod=Forward Euler  Form=Parallel  P=1  I=0  D=0.5  N=10000  InitialConditionSource=internal  InitialConditionForIntegrator=0  InitialConditionForFilter=0  ExternalReset=rising  ZeroCross=off  LimitOutput=off  UpperSaturationLimit=.5  LowerSaturationLimit=-.5  LinearizeAsGain=off  AntiWindupMode=none  Kb=1  TrackingMode=off  Kt=1  PParamMin=[]  PParamMax=[]  IParamMin=[]  IParamMax=[]  DParamMin=[]  DParamMax=[]  NParamMin=[]  NParamMax=[]  KbParamMin=[]  KbParamMax=[]  KtParamMin=[]  KtParamMax=[]  POutMin=[]  POutMax=[]  IOutMin=[]  IOutMax=[]  DOutMin=[]  DOutMax=[]  NOutMin=[]  NOutMax=[]  KbOutMin=[]  KbOutMax=[]  KtOutMin=[]  KtOutMax=[]  IntegratorOutMin=[]  IntegratorOutMax=[]  FilterOutMin=[]  FilterOutMax=[]  SumOutMin=[]  SumOutMax=[]  SumI1OutMin=[]  SumI1OutMax=[]  SumI2OutMin=[]  SumI2OutMax=[]  SumI3OutMin=[]  SumI3OutMax=[]  SumDOutMin=[]  SumDOutMax=[]  SaturationOutMin=[]  SaturationOutMax=[]  IntegratorContinuousStateAttributes=''  IntegratorStateMustResolveToSignalObject=off  IntegratorRTWStateStorageClass=Auto  FilterContinuousStateAttributes=''  FilterStateMustResolveToSignalObject=off  FilterRTWStateStorageClass=Auto
  Discrete-Time Integrator : DiscreteIntegrator  IntegratorMethod=Integration: Backward Euler  ExternalReset=either  InitialCondition=Pm0  SampleTime=-1  LimitOutput=on  UpperSaturationLimit=Tlim(2)  LowerSaturationLimit=Tlim(1)  ICPrevOutput=DiscIntNeverNeededParam  ICPrevScaledInput=DiscIntNeverNeededParam
  ENGINE Td : TransportDelay  DelayTime=Td  InitialOutput=Pm0  BufferSize=7168
  Gain K : Gain  Gain=K  SaturateOnIntegerOverflow=on  OutDataTypeStr=Inherit: Same as input  ParamDataTypeStr=Inherit: Same as input
  Mux : Mux  Inputs=2
  Mux1 : Mux  Inputs=2
  Product : Product  SaturateOnIntegerOverflow=on  InputSameDT=on  OutDataTypeStr=Inherit: Same as first input
  Product1 : Product
  Scope : Scope  NumInputPorts=4
      settings: TimeRange=6  YMin=1~-3.46945e-18~0.4075~0.105  YMax=1.02~0.13~0.435~0.135  SaveName=ScopeData2  Decimation=100
  Sum : Sum  Inputs=+-  SaturateOnIntegerOverflow=on  InputSameDT=on  OutDataTypeStr=Inherit: Same as first input
  Sum1 : Sum  Inputs=|+-
  TF3 : DiscreteTransferFcn  Numerator=T3numd  Denominator=T3dend  SampleTime=Ts  RndMeth=Nearest
  TF4 : DiscreteTransferFcn  Numerator=T4numd  Denominator=T3dend  SampleTime=Ts
  Pmec (pu) : Outport
  wires:
  Sum1/1 -> Scope/4, Pmec (pu)/1
  Product1/1 -> Damping due to pumping losses/1
  Damping due to pumping losses/1 -> Sum1/2
  w (pu)/1 -> Product/2, Mux/2, Product1/2, Product1/1, Sum/2
  Discrete PID Controller/1 -> Mux1/1, Gain K/1
  Sum/1 -> Discrete PID Controller/1
  Gain K/1 -> TF4/1
  ENGINE Td/1 -> Product/1
  wref (pu)/1 -> Mux/1, Sum/1
  Product/1 -> Sum1/1
  Discrete-Time Integrator/1 -> Scope/3, ENGINE Td/1  "Torque"
  TF3/1 -> Mux1/2, Discrete-Time Integrator/1
  TF4/1 -> TF3/1
  Reset/1 -> Discrete-Time Integrator/2, Discrete PID Controller/2
  Mux/1 -> Scope/1
  Mux1/1 -> Scope/2

== system Diesel_Genset_Test_System_80kVA/SM_Master/80kVA_Diesel_Generator/GenSet_80kVA/80kVA Generator with  Primary Controllers/Diesel Engine Speed & Voltage Control fast/Excitation1/Damping kf.s / (tf.s +1) ==
  note: link disabled
  In : Inport
  1st-Order Discrete Filter : NG_Genset_lib/NG Genset 3.5MVA/3.5MVA Generator with  Primary Controllers1/NG Engine Speed & Voltage Control fast/Excitation1/Damping kf.s // (tf.s +1)/1st-Order Discrete Filter  FilterType=Highpass  Tc=damp(2)  Ts=Ts  Initialize=on  Vac_Init=[0 0 60]  Vdc_Init=damp(1)*v0(2)/damp(2)  PlotResponse=off  param1=[1 500 0.1]
  Gain : Gain  Gain=damp(1)/damp(2)  SaturateOnIntegerOverflow=on  OutDataTypeStr=Inherit: Same as input  ParamDataTypeStr=Inherit: Same as input
  Out : Outport
  wires:
  1st-Order Discrete Filter/1 -> Out/1
  Gain/1 -> 1st-Order Discrete Filter/1
  In/1 -> Gain/1

== system Diesel_Genset_Test_System_80kVA/SM_Master/80kVA_Diesel_Generator/GenSet_80kVA/80kVA Generator with  Primary Controllers/Diesel Engine Speed & Voltage Control fast/Excitation1/Exciter  1 / (te.s + ke) ==
  note: link disabled
  In : Inport
  1st order Lowpass : NG_Genset_lib/NG Genset 3.5MVA/3.5MVA Generator with  Primary Controllers1/NG Engine Speed & Voltage Control fast/Excitation1/Exciter  1 // (te.s + ke)/1st order Lowpass  FilterType=Lowpass  Tc=exc(2)/exc(1)  Ts=Ts  Initialize=on  Vac_Init=[0.0 0 60]  Vdc_Init=v0(2)  PlotResponse=off  param1=[1 500 0.1]
  Gain : Gain  Gain=1/exc(1)  SaturateOnIntegerOverflow=on  OutDataTypeStr=Inherit: Same as input  ParamDataTypeStr=Inherit: Same as input
  Out : Outport
  wires:
  Gain/1 -> 1st order Lowpass/1
  In/1 -> Gain/1
  1st order Lowpass/1 -> Out/1

== system Diesel_Genset_Test_System_80kVA/SM_Master/80kVA_Diesel_Generator/GenSet_80kVA/80kVA Generator with  Primary Controllers/Diesel Engine Speed & Voltage Control fast/Excitation1/Main Regulator ka / (ta.s +1) ==
  note: link disabled
  In : Inport
  1st order Lowpass1 : NG_Genset_lib/NG Genset 3.5MVA/3.5MVA Generator with  Primary Controllers1/NG Engine Speed & Voltage Control fast/Excitation1/Main Regulator ka // (ta.s +1)/1st order Lowpass  FilterType=Lowpass  Tc=reg(2)  Ts=Ts  Initialize=on  Vac_Init=[0.0 0 60]  Vdc_Init=exc(1)*v0(2)  PlotResponse=off  param1=[1 500 0.1]
  Gain : Gain  Gain=reg(1)  SaturateOnIntegerOverflow=on  OutDataTypeStr=Inherit: Same as input  ParamDataTypeStr=Inherit: Same as input
  Out : Outport
  wires:
  1st order Lowpass1/1 -> Out/1
  In/1 -> Gain/1
  Gain/1 -> 1st order Lowpass1/1

== system Diesel_Genset_Test_System_80kVA/SM_Master/80kVA_Diesel_Generator/GenSet_80kVA/80kVA Generator with  Primary Controllers/Diesel Engine Speed & Voltage Control fast/Excitation1/proportional saturation ==
  Efd : Inport
  Vtf : Inport  Port=2
  Constant : Constant  Value=lim(3)
  Constant1 : Constant  Value=lim(1)
  Constant3 : Constant  Value=0
  Data Type  Conversion{,1..3} (4 alike) : DataTypeConversion  OutDataTypeStr=double  SaturateOnIntegerOverflow=on  RndMeth=Zero
  Logical Operator : Logic
  Logical Operator1 : Logic  Operator=NOT  Inputs=1
  Logical Operator2 : Logic  Operator=NOT  Inputs=1
  Product : Product  SaturateOnIntegerOverflow=on  InputSameDT=on  OutDataTypeStr=Inherit: Same as first input
  Product1 : Product  SaturateOnIntegerOverflow=on  InputSameDT=on  OutDataTypeStr=Inherit: Same as first input
  Product2 : Product  SaturateOnIntegerOverflow=on  InputSameDT=on  OutDataTypeStr=Inherit: Same as first input
  Relational Operator : RelationalOperator  Operator===  InputSameDT=on
  Relational Operator1 : RelationalOperator  Operator=<  InputSameDT=on
  Relational Operator2 : RelationalOperator  Operator=>  InputSameDT=on
  Sum : Sum  SaturateOnIntegerOverflow=on  InputSameDT=on  OutDataTypeStr=Inherit: Same as first input
  Sum1 : Sum  Inputs=+++  SaturateOnIntegerOverflow=on  InputSameDT=on  OutDataTypeStr=Inherit: Same as first input
  Vfdmax : Gain  Gain=lim(2)  SaturateOnIntegerOverflow=on  OutDataTypeStr=Inherit: Same as input  ParamDataTypeStr=Inherit: Same as input
  Vfdmax1 : Gain  Gain=lim(3)  SaturateOnIntegerOverflow=on  OutDataTypeStr=Inherit: Same as input  ParamDataTypeStr=Inherit: Same as input
  Ef : Outport  InitialOutput=0
  wires:
  Data Type  Conversion3/1 -> Vfdmax/1
  Relational Operator/1 -> Data Type  Conversion3/1
  Data Type  Conversion2/1 -> Product2/1
  Logical Operator2/1 -> Data Type  Conversion2/1
  Data Type  Conversion1/1 -> Product1/2
  Logical Operator1/1 -> Data Type  Conversion1/1
  Data Type  Conversion/1 -> Product/2
  Logical Operator/1 -> Data Type  Conversion/1
  Product1/1 -> Sum1/2
  Product2/1 -> Sum1/3
  Product/1 -> Sum1/1
  Sum1/1 -> Ef/1
  Efd/1 -> Product/1, Relational Operator1/1, Relational Operator2/1
  Constant1/1 -> Product1/1, Relational Operator2/2
  Relational Operator1/1 -> Logical Operator/2, Logical Operator2/1
  Relational Operator2/1 -> Logical Operator/1, Logical Operator1/1
  Sum/1 -> Relational Operator1/2, Product2/2
  Vfdmax1/1 -> Sum/1
  Vfdmax/1 -> Sum/2
  Constant3/1 -> Relational Operator/2
  Constant/1 -> Relational Operator/1
  Vtf/1 -> Vfdmax1/1
